simulink model "mrsObjectTrackingModel_tracking"  (R2024a)
settings: Solver=VariableStepAuto  StartTime=0.0  StopTime=inf  FixedStep=0.01  RelTol=1e-3  EnableMultiTasking=on
PreLoadFcn:
  | % Simulation parameters
  | load exampleMap
  | sampleTime = 0.05;
  | 
  | % Object Detector parameters
  | objX = 4;
  | objY = 4;
  | targetLabel = 1;
  | objLabel = 1;
  | objDetectorOffset = [0 0];
  | objDetectorAngle = 0;
  | objDetectorFOV = pi/3;
  | objDetectorRange = 5;
  | objDetectorColors = [1 0 0;0 1 0;0 0 1];
  | objDetectorMaxHits = 3;
model workspace (MAT data in the model file):
  target_position = Simulink.Parameter
  target_position.Value = [3 4]
  target_position.Complexity = 'real'
  target_position.Dimensions = [1 2]
  target_position.DataType = 'auto'
undefined symbols (not defined in the file): scanAngles
libraries: mobileRoboticsLib x7, simulink x2
settings Model: Creator=scastro  LastModifiedBy=niyu2
settings SolverCC: AlgebraicLoopSolver=TrustRegion
settings DataIOCC: LimitDataPoints=on  ReturnWorkspaceOutputs=off
settings OptimizationCC: LifeSpan=inf
settings DebuggingCC: UnconnectedInputMsg=warning  UnconnectedOutputMsg=warning  UnconnectedLineMsg=warning  AllowSymbolicDim=off  SFUnexpectedBacktrackingDiag=warning  SFNoUnconditionalDefaultTransitionDiag=warning  SFExecutionAtInitializationDiag=none  UnderSpecifiedDimensionMsg=warning  ArithmeticOperatorsInVariantConditions=warning
settings ModelReferenceCC: EnableRefExpFcnMdlSchedulingChecks=on
settings SFSimCC: SimUseLocalCustomCode=off  CustomCodeUndefinedFunction=UseInterfaceOnly
settings RTWCC: RTWUseLocalCustomCode=off  GPUComputeCapability=3.5
settings CodeAppCC: StateflowObjectComments=on
settings GRTTargetCC: TargetLangStandard=C89/C90 (ANSI)
settings ConfigComp: CovMetricSettings=dw  CovSaveCumulativeToWorkspaceVar=on  CovSaveSingleToWorkspaceVar=on  CovExternalEMLEnable=off  CovSFcnEnable=off
settings SimscapeCC: SimscapeNominalValues="[{\"value\":\"10\",\"unit\":\"V\"},{\"value\":\"1\",\"unit\":\"A\"},{\"value\":\"10\",\"unit\":\"N*m\"},{\"value\":\"10\",\"unit\":\"bar\"},{\"value\":\"100\",\"unit\":\"kJ/kg\"},{\"value\":\"1\",\"unit\":\"kW\"},{\"value\":\"300\",\"unit\":\"K\"},{\"value\":\"100\",\"unit\":\"cm^3/s\"},{\"value\":\"1\",\"unit\":\"kN\"},{\"value\":\"1\",\"unit\":\"g/cm^3\"},{\"value\":\"1\",\"unit\":\"l\"},{\"value\":\"1\",\"unit\":\"cm^2\"},{\"value\":\"60\",\"unit\":\"Hz\"}]"  SimscapeLogType=all  SimscapeLogDataHistory=10000
settings ConfigurationSet: Description=SimMechanics 2G
settings ExplorerConfigSet: InternalSimMechanicsExplorerSettings="<ExplorerConfiguration><canonicalview>default</canonicalview><AnimationSetting><BasePlaybackSpeed>1.0</BasePlaybackSpeed><PlaybackSpeedFactor>1.0</PlaybackSpeedFactor></AnimationSetting><TilePanel><TileInfo><Tiles Columns=\"1\" Count=\"1\" Rows=\"1\"><Column Weight=\"1\"/><Row Weight=\"1\"/><Tile Height=\"1\" Width=\"1\" X=\"0\" Y=\"0\"/></Tiles></TileInfo><SceneInfo><SceneViewer><BGColor><R>0.60000002384185791</R><G>0.60000002384185791</G><B>0.60000002384185791</B></BGColor><Camera><DoPerspective>off</DoPerspective><Position><X>-1.70656042355848525</X><Y>-0.974920623359631922</Y><Z>4.72930454537082046</Z></Position><Center><X>0.552860638431633689</X><Y>1.42025063411503494</Y><Z>1.4843509506914252</Z></Center><Up><X>0.664249622453917166</X><Y>0.300615402055903091</Y><Z>0.684399604848363485</Z></Up><ViewLimDist>1</ViewLimDist><YLim>2.77881717169207398</YLim><XLim>3.55928742670435394</XLim></Camera></SceneViewer></SceneInfo></TilePanel><MechEditorPanel><Cameras/><GfxPanelCameraMap/><VideoCreator><PlaybackSpeedRatio>1.0</PlaybackSpeedRatio><FrameRate>30</FrameRate><VideoFormat>Motion JPEG AVI</VideoFormat><FrameSize>auto</FrameSize></VideoCreator></MechEditorPanel></ExplorerConfiguration>"

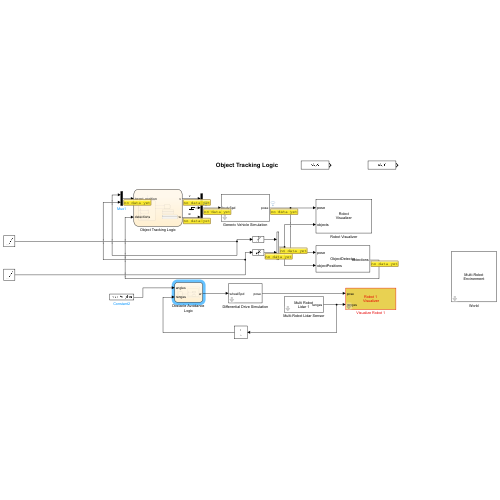
[thumbnail: Simulink's stored preview of the top-level diagram]
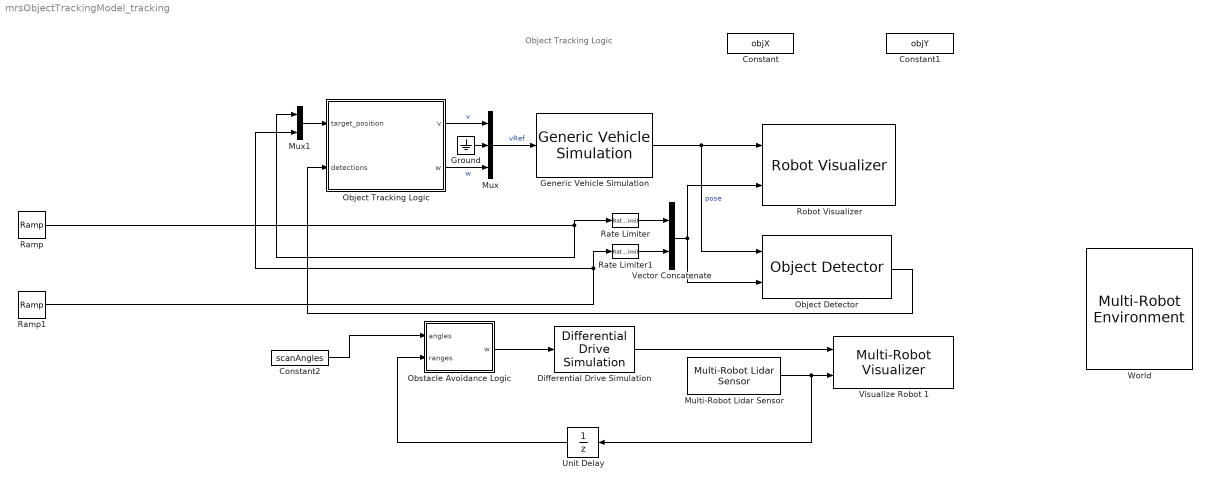
== system mrsObjectTrackingModel_tracking ==
  note: Object Tracking Logic
  Constant : Constant  Value=objX
  Constant1 : Constant  Value=objY
  Constant2 : Constant  Value=scanAngles
  Differential Drive Simulation : mobileRoboticsLib/Kinematic Models/Differential Drive/Differential Drive Simulation  wheelRadius=wheelRadius  wheelBase=robotRadius  initX=4  initY=4  initAngle=0  Ts=sampleTime
      settings: SourceProductName=Mobile Robotics Simulation Toolbox
  Generic Vehicle Simulation : mobileRoboticsLib/Utilities/Generic Vehicle Simulation  initX=2  initY=1  initAngle=0  Ts=sampleTime
      settings: SourceProductName=Mobile Robotics Simulation Toolbox
  Ground : Ground
  Multi-Robot Lidar Sensor : mobileRoboticsLib/Environments/Multi-Robot Lidar Sensor  robotIdx=1  mapName=map  sensorOffset=sensorOffset  scanAngles=scanAngles  maxRange=maxRange
      settings: SourceProductName=Mobile Robotics Simulation Toolbox
  Mux : Mux  Inputs=3
  Mux1 : Mux  Inputs=2
  Object Detector : mobileRoboticsLib/Environments/Object Detector  mapName=map  sensorOffset=objDetectorOffset  sensorAngle=objDetectorAngle  fieldOfView=objDetectorFOV  maxRange=objDetectorRange  maxDetections=objDetectorMaxHits  sampleTime=-1
      settings: SourceProductName=Mobile Robotics Simulation Toolbox
  Object Tracking Logic : Stateflow chart  TreatAsAtomicUnit=on
  Obstacle Avoidance Logic : Stateflow chart  TreatAsAtomicUnit=on
  Ramp : simulink/Sources/Ramp  slope=1  start=0  InitialOutput=2
  Ramp1 : simulink/Sources/Ramp  slope=1  start=0  InitialOutput=5
  Rate Limiter : RateLimiter  RisingSlewLimit=0.2  FallingSlewLimit=-0.5  InitialCondition=objX
  Rate Limiter1 : RateLimiter  RisingSlewLimit=0.20  InitialCondition=objX
  Robot Visualizer : mobileRoboticsLib/Environments/Robot Visualizer  Priority=99  robotRadius=0  mapName=map  showTrajectory=on  hasWaypoints=off  hasLidar=off  sensorOffset=[ 0 0 ]  scanAngles=0  hasObjDetector=on  objDetectorOffset=objDetectorOffset  objDetectorAngle=objDetectorAngle  objDetectorFOV=objDetectorFOV  objDetectorMaxRange=objDetectorRange  objectColors=objDetectorColors  objectMarkers=s
  Unit Delay : UnitDelay  SampleTime=-1  HasFrameUpgradeWarning=on
  Vector Concatenate : Concatenate  Mode=Multidimensional array  ConcatenateDimension=2
  Visualize Robot 1 : mobileRoboticsLib/Environments/Multi-Robot Visualizer  idx=1  radius=robotRadius  robotColor=[0 0 1]  showTraj=off  hasLidar=on  sensorOffset=sensorOffset  scanAngles=scanAngles  maxNumScans=0  hasObjDetector=off  objDetectorOffset=[0,0]  objDetectorAngle=0  objDetectorFOV=pi/2  objDetectorMaxRange=5  hasRobotDetector=off  robotDetectorOffset=[0,0]  robotDetectorAngle=0  robotDetectorFOV=pi/3  robotDetectorMaxRange=5  robotDetectorNumDetections=0
      settings: SourceProductName=Mobile Robotics Simulation Toolbox
  World : mobileRoboticsLib/Environments/Multi-Robot Environment  numRobots=2  mapName=map  showWaypoints=off  showObjects=off  objectColors=[1 0 0;0 1 0;0 0 1]  objectMarkers='s'  showRobotIds=on  plotSensorLines=on
      settings: SourceProductName=Mobile Robotics Simulation Toolbox
  wires:
  Generic Vehicle Simulation/1 -> Object Detector/1, Robot Visualizer/1  "pose"
  Object Tracking Logic/2(w) -> Mux/3  "w"
  Mux/1 -> Generic Vehicle Simulation/1  "vRef"
  Object Tracking Logic/1(v) -> Mux/1  "v"
  Object Detector/1 -> Object Tracking Logic/2(detections)
  Vector Concatenate/1 -> Object Detector/2, Robot Visualizer/2
  Rate Limiter/1 -> Vector Concatenate/1
  Rate Limiter1/1 -> Vector Concatenate/2
  Ground/1 -> Mux/2
  Mux1/1 -> Object Tracking Logic/1(target_position)
  Ramp1/1 -> Rate Limiter1/1, Mux1/2
  Ramp/1 -> Rate Limiter/1, Mux1/1
  Unit Delay/1 -> Obstacle Avoidance Logic/2(ranges)
  Constant2/1 -> Obstacle Avoidance Logic/1(angles)
  Differential Drive Simulation/1 -> Visualize Robot 1/1
  Multi-Robot Lidar Sensor/1 -> Unit Delay/1, Visualize Robot 1/2
  Obstacle Avoidance Logic/1(w) -> Differential Drive Simulation/1

== stateflow chart mrsObjectTrackingModel_tracking/Object Tracking Logic ==
  state TrackObject
    entry, during:
    [range,angle,valid] = findNearestObject(target_position);
    if valid
    count = 0;
    else
    count = count + 1 ;
    end
    (default) -> (junction 20)
    TrackObject -> (junction 20) [order 1]
    (junction 20) -> (junction 24) [order 1] : % Set angular speed if
        | % angle outside deadband
        | [abs(angle) > pi/24]
    (junction 20) -> (junction 30) [order 2] : {w = 0;}
    (junction 24) -> (junction 49) : % Proportional
        | % control
        | {w = 0.5*angle;}
    (junction 49) -> (junction 30)
    (junction 30) -> (junction 54)
    (junction 54) -> (junction 56) [order 1] : % Go forward if object is far
        | [range > 0]
    (junction 54) -> (junction 60) [order 2] : {v = 0;}
    (junction 56) -> (junction 58) : {v = 0.5;}
    (junction 58) -> (junction 60)
  state SeekObject
    entry:
    v = 0.1;
    w = 1;
  (default) -> TrackObject : {
      | count = 0;
      | range = 0;
      | angle = 0;
      | }
  TrackObject -> SeekObject [order 1] : [count >= 20]
  SeekObject -> TrackObject : [~isempty(detections)]
  data: dist function_output; ang function_output; flag function_output; label function_input; dist function_output; ang function_output; flag function_output; target_position function_input; target_position input; detections input size=[objDetectorMaxHits,3]; v output; w output; angle local; range local; count local; valid local
  function [dist,ang,flag] = findValidObject(label):
    | function [dist,ang,flag] = findValidObject(label)
    | % Finds the distance (dist) and angle (ang) of the nearest valid
    | % object detected. If an object is found, the (flag) output is true.
    | 
    | % Initialize
    | flag = false;
    | dist = 0;
    | ang = 0;
    | 
    | if ~isempty(detections)
    |     % Loop through all detections
    |     for idx = 1:size(detections,1)
    |         % If a detection matching the target label is found, 
    |         % return it and set the valid flag to true.
    |         if detections(idx,3) == label
    |             dist = detections(idx,1);
    |             ang  = detections(idx,2);
    |             flag = true;
    |             return; 
    |         end
    |     end
    | end
  function [dist, ang, flag] = findNearestObject(target_position):
    | function [dist, ang, flag] = findNearestObject(target_position)
    | % Finds the distance (dist) and angle (ang) of the nearest object to the 
    | % target_position. If an object is found, the (flag) output is true.
    | 
    | % Initialize
    | flag = false;
    | dist = Inf; % Set to Inf initially to find the minimum distance
    | ang = 0;
    | 
    | if ~isempty(detections)==true
    |     % Loop through all detections
    |     for idx = 1:size(detections,1)
    |         % Get the position of the current detection
    |         object_position = [detections(idx,1), detections(idx,2)];
    |         
    |         % Calculate the Euclidean distance to the target position
    |         current_dist = norm([object_position(1) - target_position(1), object_position(2) - target_position(2)]);
    |         
    |         % If this is the nearest object so far, update the distance, angle, and flag
    |         if current_dist < dist
    |             dist = current_dist;
    |             ang = atan2(object_position(2) - target_position(2), object_position(1) - target_position(1));
    |             flag = true;
    |         end
    |     end
    | end
    | end

== stateflow chart mrsObjectTrackingModel_tracking/Obstacle Avoidance Logic ==
  state MainState [parallel]
    en,du:
    validIdx = ~isnan(ranges);
    validRanges = ranges(validIdx);
    validAngles = angles(validIdx);
    settings: executionOrder=1
    state Turn
      en,du:
      avgAngle = mean(validAngles./validRanges);
      state Left
        en, du:
        w = [0;12.5];
      state Right
        en, du:
        w = [12.5;0];
      (default) -> (junction 39)
      (junction 39) -> Left [order 1] : [avgAngle < 0]
      (junction 39) -> (junction 43) [order 2]
      Left -> Right : [after(1,sec) && ...
          | avgAngle > 0]
      Right -> Left : [after(1,sec) && ...
          | avgAngle < 0]
      (junction 43) -> Right
    state GoStraight
      en:
      w = [25; 25];
    (default) -> GoStraight
    GoStraight -> Turn : [any(validRanges<=1)]
    Turn -> GoStraight : [all(validRanges>1)]
  data: angles input; w output; ranges input; validRanges local size=numel(scanAngles); validIdx local; validAngles local size=numel(scanAngles); avgAngle local
